simulink model "gm_hybrid_lht"  (R2019b)
settings: Solver=FixedStepDiscrete  StartTime=0.0  StopTime=inf  FixedStep=1/120e6  RelTol=1e-3
undefined symbols (not defined in the file or in its folder): bt, height, nTheta, width
libraries: hdlsllib x42, simulink x32, hdlmdlgenlib x7, dspsrcs4 x1
(part 3 of 3)

== system gm_hybrid_lht/Hybrid LHT/Hybrid LHT Accumulator/Accumulator with Switches/Accumulator_instance2/Block RAM/Simple Dual Port RAM Generator ==
  wr_data : Inport  OutDataTypeStr=fixdt(0, 36, 0)  PortDimensions=1  SampleTime=8.33333333333333e-09
  wr_addr : Inport  Port=2  OutDataTypeStr=fixdt(0, 10, 0)  PortDimensions=1  SampleTime=8.33333333333333e-09
  wr_en : Inport  Port=3  OutDataTypeStr=boolean  PortDimensions=1  SampleTime=8.33333333333333e-09
  rd_addr : Inport  Port=4  OutDataTypeStr=fixdt(0, 10, 0)  PortDimensions=1  SampleTime=8.33333333333333e-09
  rd_address : hdlsllib/Logic and Bit Operations/Bit Slice  lidx=9  ridx=0
      settings: SourceProductName=Simulink  SourceProductBaseCode=SL
  simple_ram_0 : hdlsllib/HDL RAMs/Simple Dual Port RAM  ram_size=10
      settings: SourceProductName=Simulink  SourceProductBaseCode=SL
  wr_address : hdlsllib/Logic and Bit Operations/Bit Slice  lidx=9  ridx=0
      settings: SourceProductName=Simulink  SourceProductBaseCode=SL
  rd_data : Outport
  wires:
  rd_addr/1 -> rd_address/1
  wr_en/1 -> simple_ram_0/3
  wr_addr/1 -> wr_address/1
  wr_data/1 -> simple_ram_0/1
  rd_address/1 -> simple_ram_0/4
  simple_ram_0/1 -> rd_data/1
  wr_address/1 -> simple_ram_0/2

== system gm_hybrid_lht/Hybrid LHT/Hybrid LHT Accumulator/Accumulator with Switches/Accumulator_instance3/Block RAM/Simple Dual Port RAM Generator ==
  wr_data : Inport  OutDataTypeStr=fixdt(0, 36, 0)  PortDimensions=1  SampleTime=8.33333333333333e-09
  wr_addr : Inport  Port=2  OutDataTypeStr=fixdt(0, 10, 0)  PortDimensions=1  SampleTime=8.33333333333333e-09
  wr_en : Inport  Port=3  OutDataTypeStr=boolean  PortDimensions=1  SampleTime=8.33333333333333e-09
  rd_addr : Inport  Port=4  OutDataTypeStr=fixdt(0, 10, 0)  PortDimensions=1  SampleTime=8.33333333333333e-09
  rd_address : hdlsllib/Logic and Bit Operations/Bit Slice  lidx=9  ridx=0
      settings: SourceProductName=Simulink  SourceProductBaseCode=SL
  simple_ram_0 : hdlsllib/HDL RAMs/Simple Dual Port RAM  ram_size=10
      settings: SourceProductName=Simulink  SourceProductBaseCode=SL
  wr_address : hdlsllib/Logic and Bit Operations/Bit Slice  lidx=9  ridx=0
      settings: SourceProductName=Simulink  SourceProductBaseCode=SL
  rd_data : Outport
  wires:
  rd_addr/1 -> rd_address/1
  wr_en/1 -> simple_ram_0/3
  wr_addr/1 -> wr_address/1
  wr_data/1 -> simple_ram_0/1
  rd_address/1 -> simple_ram_0/4
  simple_ram_0/1 -> rd_data/1
  wr_address/1 -> simple_ram_0/2

== system gm_hybrid_lht/Hybrid LHT/Hybrid LHT Accumulator/Accumulator with Switches/Accumulator_instance4/Block RAM/Simple Dual Port RAM Generator ==
  wr_data : Inport  OutDataTypeStr=fixdt(0, 36, 0)  PortDimensions=1  SampleTime=8.33333333333333e-09
  wr_addr : Inport  Port=2  OutDataTypeStr=fixdt(0, 10, 0)  PortDimensions=1  SampleTime=8.33333333333333e-09
  wr_en : Inport  Port=3  OutDataTypeStr=boolean  PortDimensions=1  SampleTime=8.33333333333333e-09
  rd_addr : Inport  Port=4  OutDataTypeStr=fixdt(0, 10, 0)  PortDimensions=1  SampleTime=8.33333333333333e-09
  rd_address : hdlsllib/Logic and Bit Operations/Bit Slice  lidx=9  ridx=0
      settings: SourceProductName=Simulink  SourceProductBaseCode=SL
  simple_ram_0 : hdlsllib/HDL RAMs/Simple Dual Port RAM  ram_size=10
      settings: SourceProductName=Simulink  SourceProductBaseCode=SL
  wr_address : hdlsllib/Logic and Bit Operations/Bit Slice  lidx=9  ridx=0
      settings: SourceProductName=Simulink  SourceProductBaseCode=SL
  rd_data : Outport
  wires:
  rd_addr/1 -> rd_address/1
  wr_en/1 -> simple_ram_0/3
  wr_addr/1 -> wr_address/1
  wr_data/1 -> simple_ram_0/1
  rd_address/1 -> simple_ram_0/4
  simple_ram_0/1 -> rd_data/1
  wr_address/1 -> simple_ram_0/2

== system gm_hybrid_lht/Hybrid LHT/Hybrid LHT Accumulator/Accumulator with Switches/Accumulator_instance5/Block RAM/Simple Dual Port RAM Generator ==
  wr_data : Inport  OutDataTypeStr=fixdt(0, 36, 0)  PortDimensions=1  SampleTime=8.33333333333333e-09
  wr_addr : Inport  Port=2  OutDataTypeStr=fixdt(0, 10, 0)  PortDimensions=1  SampleTime=8.33333333333333e-09
  wr_en : Inport  Port=3  OutDataTypeStr=boolean  PortDimensions=1  SampleTime=8.33333333333333e-09
  rd_addr : Inport  Port=4  OutDataTypeStr=fixdt(0, 10, 0)  PortDimensions=1  SampleTime=8.33333333333333e-09
  rd_address : hdlsllib/Logic and Bit Operations/Bit Slice  lidx=9  ridx=0
      settings: SourceProductName=Simulink  SourceProductBaseCode=SL
  simple_ram_0 : hdlsllib/HDL RAMs/Simple Dual Port RAM  ram_size=10
      settings: SourceProductName=Simulink  SourceProductBaseCode=SL
  wr_address : hdlsllib/Logic and Bit Operations/Bit Slice  lidx=9  ridx=0
      settings: SourceProductName=Simulink  SourceProductBaseCode=SL
  rd_data : Outport
  wires:
  rd_addr/1 -> rd_address/1
  wr_en/1 -> simple_ram_0/3
  wr_addr/1 -> wr_address/1
  wr_data/1 -> simple_ram_0/1
  rd_address/1 -> simple_ram_0/4
  simple_ram_0/1 -> rd_data/1
  wr_address/1 -> simple_ram_0/2

== system gm_hybrid_lht/Hybrid LHT/Hybrid LHT Accumulator/Accumulator with Switches/Accumulator_instance6/Block RAM/Simple Dual Port RAM Generator ==
  wr_data : Inport  OutDataTypeStr=fixdt(0, 36, 0)  PortDimensions=1  SampleTime=8.33333333333333e-09
  wr_addr : Inport  Port=2  OutDataTypeStr=fixdt(0, 10, 0)  PortDimensions=1  SampleTime=8.33333333333333e-09
  wr_en : Inport  Port=3  OutDataTypeStr=boolean  PortDimensions=1  SampleTime=8.33333333333333e-09
  rd_addr : Inport  Port=4  OutDataTypeStr=fixdt(0, 10, 0)  PortDimensions=1  SampleTime=8.33333333333333e-09
  rd_address : hdlsllib/Logic and Bit Operations/Bit Slice  lidx=9  ridx=0
      settings: SourceProductName=Simulink  SourceProductBaseCode=SL
  simple_ram_0 : hdlsllib/HDL RAMs/Simple Dual Port RAM  ram_size=10
      settings: SourceProductName=Simulink  SourceProductBaseCode=SL
  wr_address : hdlsllib/Logic and Bit Operations/Bit Slice  lidx=9  ridx=0
      settings: SourceProductName=Simulink  SourceProductBaseCode=SL
  rd_data : Outport
  wires:
  rd_addr/1 -> rd_address/1
  wr_en/1 -> simple_ram_0/3
  wr_addr/1 -> wr_address/1
  wr_data/1 -> simple_ram_0/1
  rd_address/1 -> simple_ram_0/4
  simple_ram_0/1 -> rd_data/1
  wr_address/1 -> simple_ram_0/2

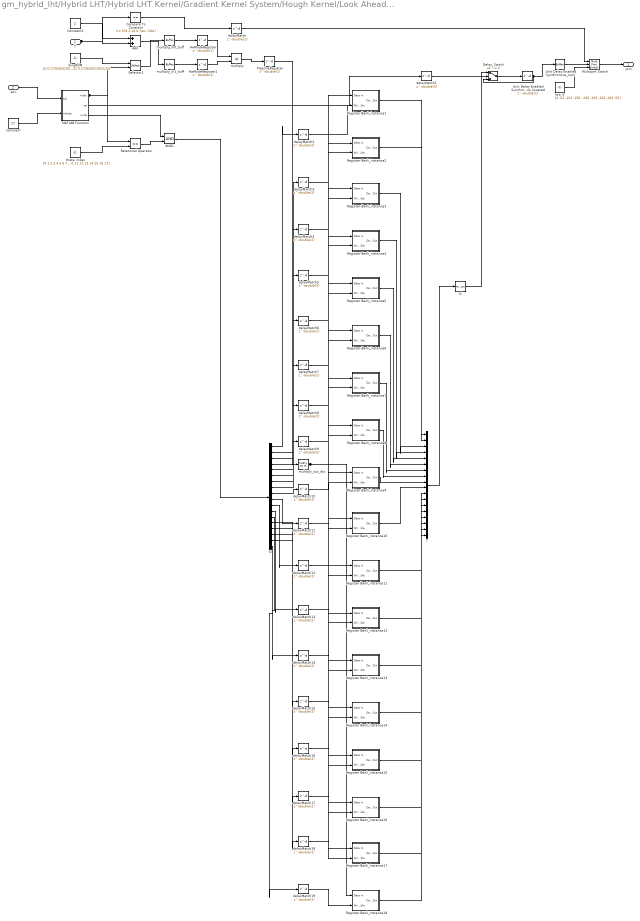
== system gm_hybrid_lht/Hybrid LHT/Hybrid LHT Kernel/Gradient Kernel System/Hough Kernel/Look Ahead Hough/Look Ahead Hough ==
  Y : Inport  OutDataTypeStr=fixdt(1, 10, 0)  PortDimensions=1  SampleTime=8.33333333333333e-09
  eol : Inport  Port=2  OutDataTypeStr=boolean  PortDimensions=1  SampleTime=8.33333333333333e-09
  AND1 : Logic  AllPortsSameDT=off  OutDataTypeStr=boolean  SampleTime=8.33333333333333e-09
  Add : Sum  AccumDataTypeStr=fixdt(1, 11, 0)  OutDataTypeStr=fixdt(1, 10, 0)  SampleTime=8.33333333333333e-09
  Compare To Constant : simulink/Logic and Bit Operations/Compare To Constant  relop===  const=fi(0,1,10,0,'hex','2d4')  OutDataTypeStr=boolean
  Constant : Constant  Value=17  OutDataTypeStr=fixdt(0, 5, 0)  SampleTime=-1
  Constant1 : Constant  OutDataTypeStr=fixdt(1, 10, 0)  SampleTime=-1
  Delay_Switch : Switch  Criteria=u2 ~= 0  Threshold=double(0)  OutDataTypeStr=fixdt(1, 10, 0)  SampleTime=8.33333333333333e-09
  HwModeRegister : Delay  DelayLength=double(1)  InitialCondition=0  SampleTime=8.33333333333333e-09
  HwModeRegister1 : Delay  DelayLength=double(1)  InitialCondition=0  SampleTime=8.33333333333333e-09
  MATLAB Function : Subsystem
  Multiport Switch : MultiPortSwitch  DataPortOrder=Zero-based contiguous  Inputs=2  DiagnosticForDefault=None  zeroidx=on  OutDataTypeStr=fixdt(1, 10, 0)  SampleTime=8.33333333333333e-09
  PipelineRegister : Delay  DelayLength=double(1)  InitialCondition=0  SampleTime=8.33333333333333e-09
  Register Bank_instance1 : Subsystem
  Register Bank_instance10 : Subsystem
  Register Bank_instance11 : Subsystem
  Register Bank_instance12 : Subsystem
  Register Bank_instance13 : Subsystem
  Register Bank_instance14 : Subsystem
  Register Bank_instance15 : Subsystem
  Register Bank_instance16 : Subsystem
  Register Bank_instance17 : Subsystem
  Register Bank_instance18 : Subsystem
  Register Bank_instance2 : Subsystem
  Register Bank_instance3 : Subsystem
  Register Bank_instance4 : Subsystem
  Register Bank_instance5 : Subsystem
  Register Bank_instance6 : Subsystem
  Register Bank_instance7 : Subsystem
  Register Bank_instance8 : Subsystem
  Register Bank_instance9 : Subsystem
  Relational Operator : RelationalOperator  Operator===  OutDataTypeStr=boolean  SampleTime=8.33333333333333e-09  RndMeth=Nearest
  Selector1 : Selector  NumberOfDimensions=2  IndexMode=Zero-based  SampleTime=8.33333333333333e-09  IndexOptions=Index vector (dialog),Index vector (port)  Indices=double(0),double(1)  OutputSizes=double(1),double(1)
  SineROM : Constant  Value=[0 0.17364501953125 0.342041015625 0.5 0.64276123046875 0.76605224609375 0.86602783203125 0.939697265625 0.98480224609375 1 0.98480224609375 0.939697265625 0.86602783203125 0.76605224609375 0.64276123046875 0.5 0.342041015625 0.17364501953125]  VectorParams1D=off  OutDataTypeStr=fixdt(1, 16, 14)  SampleTime=-1
  Unit Delay Enabled Synchronous_lowered : Delay  DelayLength=double(1)  InitialCondition=0  SampleTime=8.33333333333333e-09
  Unit Delay Enabled Synchronous_out1 : hdlmdlgenlib/Buffer
      settings: SourceProductName=Simulink  SourceProductBaseCode=SL
  delayMatch{,1..19} (20 alike) : Delay  DelayLength=double(2)  InitialCondition=0  SampleTime=8.33333333333333e-09
  multiply : Product  Inputs=**  OutDataTypeStr=fixdt(1, 26, 14)  SampleTime=8.33333333333333e-09
  multiply_in0_buff : hdlmdlgenlib/Buffer
      settings: SourceProductName=Simulink  SourceProductBaseCode=SL
  multiply_in1_buff : hdlmdlgenlib/Buffer
      settings: SourceProductName=Simulink  SourceProductBaseCode=SL
  multiply_out_dtc : DataTypeConversion  OutDataTypeStr=fixdt(1, 10, 0)  RndMeth=Round  SampleTime=8.33333333333333e-09
  row_0 : Constant  Value=[0 -52 -103 -150 -193 -230 -260 -282 -295 -300 -295 -282 -260 -230 -193 -150 -103 -52]  VectorParams1D=off  OutDataTypeStr=fixdt(1, 10, 0)  SampleTime=-1
  t : Concatenate  NumInputs=18
  t1 : Reshape  OutputDimensionality=Row vector (2-D)
  t2 : Demux  Outputs=18
  theta_index : Constant  Value=[0 1 2 3 4 5 6 7 8 9 10 11 12 13 14 15 16 17]  VectorParams1D=off  OutDataTypeStr=uint8  SampleTime=-1
  ysin : Outport  VectorParamsAs1DForOutWhenUnconnected=off
  wires:
  Constant/1 -> MATLAB Function/2(ntheta)
  Constant1/1 -> Add/1
  MATLAB Function/1(index) -> Relational Operator/1, Selector1/2
  MATLAB Function/3(write) -> AND1/1
  Multiport Switch/1 -> ysin/1
  Relational Operator/1 -> AND1/2
  SineROM/1 -> Selector1/1
  row_0/1 -> Multiport Switch/3
  theta_index/1 -> Relational Operator/2
  Y/1 -> Add/2, Compare To Constant/1
  eol/1 -> MATLAB Function/1(eol)
  MATLAB Function/2(sel) -> delayMatch1/1
  Compare To Constant/1 -> delayMatch/1
  delayMatch/1 -> Multiport Switch/1
  Unit Delay Enabled Synchronous_out1/1 -> Multiport Switch/2
  Unit Delay Enabled Synchronous_lowered/1 -> Delay_Switch/3, Unit Delay Enabled Synchronous_out1/1
  delayMatch1/1 -> Delay_Switch/2
  Delay_Switch/1 -> Unit Delay Enabled Synchronous_lowered/1
  t1/1 -> Delay_Switch/1
  delayMatch2/1 -> Register Bank_instance1/2(Write Enable)
  delayMatch3/1 -> Register Bank_instance2/2(Write Enable)
  Register Bank_instance3/1(Data Out) -> t/3
  delayMatch4/1 -> Register Bank_instance3/2(Write Enable)
  Register Bank_instance4/1(Data Out) -> t/4
  delayMatch5/1 -> Register Bank_instance4/2(Write Enable)
  Register Bank_instance5/1(Data Out) -> t/5
  delayMatch6/1 -> Register Bank_instance5/2(Write Enable)
  Register Bank_instance6/1(Data Out) -> t/6
  delayMatch7/1 -> Register Bank_instance6/2(Write Enable)
  Register Bank_instance7/1(Data Out) -> t/7
  delayMatch8/1 -> Register Bank_instance7/2(Write Enable)
  Register Bank_instance8/1(Data Out) -> t/8
  delayMatch9/1 -> Register Bank_instance8/2(Write Enable)
  Register Bank_instance9/1(Data Out) -> t/9
  delayMatch10/1 -> Register Bank_instance9/2(Write Enable)
  Register Bank_instance10/1(Data Out) -> t/10
  delayMatch11/1 -> Register Bank_instance10/2(Write Enable)
  Register Bank_instance11/1(Data Out) -> t/11
  delayMatch12/1 -> Register Bank_instance11/2(Write Enable)
  Register Bank_instance12/1(Data Out) -> t/12
  delayMatch13/1 -> Register Bank_instance12/2(Write Enable)
  Register Bank_instance13/1(Data Out) -> t/13
  delayMatch14/1 -> Register Bank_instance13/2(Write Enable)
  Register Bank_instance14/1(Data Out) -> t/14
  delayMatch15/1 -> Register Bank_instance14/2(Write Enable)
  Register Bank_instance15/1(Data Out) -> t/15
  delayMatch16/1 -> Register Bank_instance15/2(Write Enable)
  Register Bank_instance16/1(Data Out) -> t/16
  delayMatch17/1 -> Register Bank_instance16/2(Write Enable)
  Register Bank_instance17/1(Data Out) -> t/17
  delayMatch18/1 -> Register Bank_instance17/2(Write Enable)
  AND1/1 -> t2/1
  t2/1 -> delayMatch2/1
  t2/2 -> delayMatch3/1
  t2/3 -> delayMatch4/1
  t2/4 -> delayMatch5/1
  t2/5 -> delayMatch6/1
  t2/6 -> delayMatch7/1
  t2/7 -> delayMatch8/1
  t2/8 -> delayMatch9/1
  t2/9 -> delayMatch10/1
  t2/10 -> delayMatch11/1
  t2/11 -> delayMatch12/1
  t2/12 -> delayMatch13/1
  t2/13 -> delayMatch14/1
  t2/14 -> delayMatch15/1
  t2/15 -> delayMatch16/1
  t2/16 -> delayMatch17/1
  t2/17 -> delayMatch18/1
  t2/18 -> delayMatch19/1
  delayMatch19/1 -> Register Bank_instance18/2(Write Enable)
  Register Bank_instance18/1(Data Out) -> t/18
  Selector1/1 -> multiply_in0_buff/1
  Add/1 -> multiply_in1_buff/1
  PipelineRegister/1 -> multiply_out_dtc/1
  multiply_out_dtc/1 -> Register Bank_instance18/1(Data In), Register Bank_instance17/1(Data In), Register Bank_instance16/1(Data In), Register Bank_instance15/1(Data In), Register Bank_instance14/1(Data In), Register Bank_instance13/1(Data In), Register Bank_instance12/1(Data In), Register Bank_instance11/1(Data In), Register Bank_instance10/1(Data In), Register Bank_instance9/1(Data In), Register Bank_instance8/1(Data In), Register Bank_instance7/1(Data In), Register Bank_instance6/1(Data In), Register Bank_instance5/1(Data In), Register Bank_instance4/1(Data In), Register Bank_instance3/1(Data In), Register Bank_instance2/1(Data In), Register Bank_instance1/1(Data In)
  Register Bank_instance2/1(Data Out) -> t/2
  Register Bank_instance1/1(Data Out) -> t/1
  t/1 -> t1/1
  multiply/1 -> PipelineRegister/1
  HwModeRegister/1 -> multiply/1
  HwModeRegister1/1 -> multiply/2
  multiply_in0_buff/1 -> HwModeRegister/1
  multiply_in1_buff/1 -> HwModeRegister1/1

== system gm_hybrid_lht/Hybrid LHT/Hybrid LHT Kernel/Gradient Kernel System/Hough Kernel/Look Ahead Hough/Look Ahead Hough/MATLAB Function ==
  eol : Inport  OutDataTypeStr=boolean  PortDimensions=1  SampleTime=8.33333333333333e-09
  ntheta : Inport  Port=2  OutDataTypeStr=fixdt(0, 5, 0)  PortDimensions=1  SampleTime=8.33333333333333e-09
  MATLAB Function : MATLAB Function  TreatAsAtomicUnit=on
  index : Outport  VectorParamsAs1DForOutWhenUnconnected=off
  sel : Outport  Port=2  VectorParamsAs1DForOutWhenUnconnected=off
  write : Outport  Port=3  VectorParamsAs1DForOutWhenUnconnected=off
  wires:
  MATLAB Function/1(index) -> index/1
  MATLAB Function/2(sel) -> sel/1
  MATLAB Function/3(write) -> write/1
  eol/1 -> MATLAB Function/1(eol)
  ntheta/1 -> MATLAB Function/2(ntheta)

== system gm_hybrid_lht/Hybrid LHT/Hybrid LHT Kernel/Gradient Kernel System/Hough Kernel/Look Ahead Hough/Look Ahead Hough/Register Bank_instance1 ==
  Data In : Inport  OutDataTypeStr=fixdt(1, 10, 0)  PortDimensions=1  SampleTime=8.33333333333333e-09
  Write Enable : Inport  Port=2  OutDataTypeStr=boolean  PortDimensions=1  SampleTime=8.33333333333333e-09
  Delay_Switch : Switch  Criteria=u2 ~= 0  Threshold=double(0)  OutDataTypeStr=fixdt(1, 10, 0)  SampleTime=8.33333333333333e-09
  Unit Delay Enabled Synchronous_lowered : Delay  DelayLength=double(1)  InitialCondition=0  SampleTime=8.33333333333333e-09
  Data Out : Outport
  wires:
  Delay_Switch/1 -> Unit Delay Enabled Synchronous_lowered/1
  Write Enable/1 -> Delay_Switch/2
  Data In/1 -> Delay_Switch/1
  Unit Delay Enabled Synchronous_lowered/1 -> Delay_Switch/3, Data Out/1

== system gm_hybrid_lht/Hybrid LHT/Hybrid LHT Kernel/Gradient Kernel System/Hough Kernel/Look Ahead Hough/Look Ahead Hough/Register Bank_instance10 ==
  Data In : Inport  OutDataTypeStr=fixdt(1, 10, 0)  PortDimensions=1  SampleTime=8.33333333333333e-09
  Write Enable : Inport  Port=2  OutDataTypeStr=boolean  PortDimensions=1  SampleTime=8.33333333333333e-09
  Delay_Switch : Switch  Criteria=u2 ~= 0  Threshold=double(0)  OutDataTypeStr=fixdt(1, 10, 0)  SampleTime=8.33333333333333e-09
  Unit Delay Enabled Synchronous_lowered : Delay  DelayLength=double(1)  InitialCondition=0  SampleTime=8.33333333333333e-09
  Data Out : Outport
  wires:
  Delay_Switch/1 -> Unit Delay Enabled Synchronous_lowered/1
  Write Enable/1 -> Delay_Switch/2
  Data In/1 -> Delay_Switch/1
  Unit Delay Enabled Synchronous_lowered/1 -> Delay_Switch/3, Data Out/1

== system gm_hybrid_lht/Hybrid LHT/Hybrid LHT Kernel/Gradient Kernel System/Hough Kernel/Look Ahead Hough/Look Ahead Hough/Register Bank_instance11 ==
  Data In : Inport  OutDataTypeStr=fixdt(1, 10, 0)  PortDimensions=1  SampleTime=8.33333333333333e-09
  Write Enable : Inport  Port=2  OutDataTypeStr=boolean  PortDimensions=1  SampleTime=8.33333333333333e-09
  Delay_Switch : Switch  Criteria=u2 ~= 0  Threshold=double(0)  OutDataTypeStr=fixdt(1, 10, 0)  SampleTime=8.33333333333333e-09
  Unit Delay Enabled Synchronous_lowered : Delay  DelayLength=double(1)  InitialCondition=0  SampleTime=8.33333333333333e-09
  Data Out : Outport
  wires:
  Delay_Switch/1 -> Unit Delay Enabled Synchronous_lowered/1
  Write Enable/1 -> Delay_Switch/2
  Data In/1 -> Delay_Switch/1
  Unit Delay Enabled Synchronous_lowered/1 -> Delay_Switch/3, Data Out/1

== system gm_hybrid_lht/Hybrid LHT/Hybrid LHT Kernel/Gradient Kernel System/Hough Kernel/Look Ahead Hough/Look Ahead Hough/Register Bank_instance12 ==
  Data In : Inport  OutDataTypeStr=fixdt(1, 10, 0)  PortDimensions=1  SampleTime=8.33333333333333e-09
  Write Enable : Inport  Port=2  OutDataTypeStr=boolean  PortDimensions=1  SampleTime=8.33333333333333e-09
  Delay_Switch : Switch  Criteria=u2 ~= 0  Threshold=double(0)  OutDataTypeStr=fixdt(1, 10, 0)  SampleTime=8.33333333333333e-09
  Unit Delay Enabled Synchronous_lowered : Delay  DelayLength=double(1)  InitialCondition=0  SampleTime=8.33333333333333e-09
  Data Out : Outport
  wires:
  Delay_Switch/1 -> Unit Delay Enabled Synchronous_lowered/1
  Write Enable/1 -> Delay_Switch/2
  Data In/1 -> Delay_Switch/1
  Unit Delay Enabled Synchronous_lowered/1 -> Delay_Switch/3, Data Out/1

== system gm_hybrid_lht/Hybrid LHT/Hybrid LHT Kernel/Gradient Kernel System/Hough Kernel/Look Ahead Hough/Look Ahead Hough/Register Bank_instance13 ==
  Data In : Inport  OutDataTypeStr=fixdt(1, 10, 0)  PortDimensions=1  SampleTime=8.33333333333333e-09
  Write Enable : Inport  Port=2  OutDataTypeStr=boolean  PortDimensions=1  SampleTime=8.33333333333333e-09
  Delay_Switch : Switch  Criteria=u2 ~= 0  Threshold=double(0)  OutDataTypeStr=fixdt(1, 10, 0)  SampleTime=8.33333333333333e-09
  Unit Delay Enabled Synchronous_lowered : Delay  DelayLength=double(1)  InitialCondition=0  SampleTime=8.33333333333333e-09
  Data Out : Outport
  wires:
  Delay_Switch/1 -> Unit Delay Enabled Synchronous_lowered/1
  Write Enable/1 -> Delay_Switch/2
  Data In/1 -> Delay_Switch/1
  Unit Delay Enabled Synchronous_lowered/1 -> Delay_Switch/3, Data Out/1

== system gm_hybrid_lht/Hybrid LHT/Hybrid LHT Kernel/Gradient Kernel System/Hough Kernel/Look Ahead Hough/Look Ahead Hough/Register Bank_instance14 ==
  Data In : Inport  OutDataTypeStr=fixdt(1, 10, 0)  PortDimensions=1  SampleTime=8.33333333333333e-09
  Write Enable : Inport  Port=2  OutDataTypeStr=boolean  PortDimensions=1  SampleTime=8.33333333333333e-09
  Delay_Switch : Switch  Criteria=u2 ~= 0  Threshold=double(0)  OutDataTypeStr=fixdt(1, 10, 0)  SampleTime=8.33333333333333e-09
  Unit Delay Enabled Synchronous_lowered : Delay  DelayLength=double(1)  InitialCondition=0  SampleTime=8.33333333333333e-09
  Data Out : Outport
  wires:
  Delay_Switch/1 -> Unit Delay Enabled Synchronous_lowered/1
  Write Enable/1 -> Delay_Switch/2
  Data In/1 -> Delay_Switch/1
  Unit Delay Enabled Synchronous_lowered/1 -> Delay_Switch/3, Data Out/1

== system gm_hybrid_lht/Hybrid LHT/Hybrid LHT Kernel/Gradient Kernel System/Hough Kernel/Look Ahead Hough/Look Ahead Hough/Register Bank_instance15 ==
  Data In : Inport  OutDataTypeStr=fixdt(1, 10, 0)  PortDimensions=1  SampleTime=8.33333333333333e-09
  Write Enable : Inport  Port=2  OutDataTypeStr=boolean  PortDimensions=1  SampleTime=8.33333333333333e-09
  Delay_Switch : Switch  Criteria=u2 ~= 0  Threshold=double(0)  OutDataTypeStr=fixdt(1, 10, 0)  SampleTime=8.33333333333333e-09
  Unit Delay Enabled Synchronous_lowered : Delay  DelayLength=double(1)  InitialCondition=0  SampleTime=8.33333333333333e-09
  Data Out : Outport
  wires:
  Delay_Switch/1 -> Unit Delay Enabled Synchronous_lowered/1
  Write Enable/1 -> Delay_Switch/2
  Data In/1 -> Delay_Switch/1
  Unit Delay Enabled Synchronous_lowered/1 -> Delay_Switch/3, Data Out/1

== system gm_hybrid_lht/Hybrid LHT/Hybrid LHT Kernel/Gradient Kernel System/Hough Kernel/Look Ahead Hough/Look Ahead Hough/Register Bank_instance16 ==
  Data In : Inport  OutDataTypeStr=fixdt(1, 10, 0)  PortDimensions=1  SampleTime=8.33333333333333e-09
  Write Enable : Inport  Port=2  OutDataTypeStr=boolean  PortDimensions=1  SampleTime=8.33333333333333e-09
  Delay_Switch : Switch  Criteria=u2 ~= 0  Threshold=double(0)  OutDataTypeStr=fixdt(1, 10, 0)  SampleTime=8.33333333333333e-09
  Unit Delay Enabled Synchronous_lowered : Delay  DelayLength=double(1)  InitialCondition=0  SampleTime=8.33333333333333e-09
  Data Out : Outport
  wires:
  Delay_Switch/1 -> Unit Delay Enabled Synchronous_lowered/1
  Write Enable/1 -> Delay_Switch/2
  Data In/1 -> Delay_Switch/1
  Unit Delay Enabled Synchronous_lowered/1 -> Delay_Switch/3, Data Out/1

== system gm_hybrid_lht/Hybrid LHT/Hybrid LHT Kernel/Gradient Kernel System/Hough Kernel/Look Ahead Hough/Look Ahead Hough/Register Bank_instance17 ==
  Data In : Inport  OutDataTypeStr=fixdt(1, 10, 0)  PortDimensions=1  SampleTime=8.33333333333333e-09
  Write Enable : Inport  Port=2  OutDataTypeStr=boolean  PortDimensions=1  SampleTime=8.33333333333333e-09
  Delay_Switch : Switch  Criteria=u2 ~= 0  Threshold=double(0)  OutDataTypeStr=fixdt(1, 10, 0)  SampleTime=8.33333333333333e-09
  Unit Delay Enabled Synchronous_lowered : Delay  DelayLength=double(1)  InitialCondition=0  SampleTime=8.33333333333333e-09
  Data Out : Outport
  wires:
  Delay_Switch/1 -> Unit Delay Enabled Synchronous_lowered/1
  Write Enable/1 -> Delay_Switch/2
  Data In/1 -> Delay_Switch/1
  Unit Delay Enabled Synchronous_lowered/1 -> Delay_Switch/3, Data Out/1

== system gm_hybrid_lht/Hybrid LHT/Hybrid LHT Kernel/Gradient Kernel System/Hough Kernel/Look Ahead Hough/Look Ahead Hough/Register Bank_instance18 ==
  Data In : Inport  OutDataTypeStr=fixdt(1, 10, 0)  PortDimensions=1  SampleTime=8.33333333333333e-09
  Write Enable : Inport  Port=2  OutDataTypeStr=boolean  PortDimensions=1  SampleTime=8.33333333333333e-09
  Delay_Switch : Switch  Criteria=u2 ~= 0  Threshold=double(0)  OutDataTypeStr=fixdt(1, 10, 0)  SampleTime=8.33333333333333e-09
  Unit Delay Enabled Synchronous_lowered : Delay  DelayLength=double(1)  InitialCondition=0  SampleTime=8.33333333333333e-09
  Data Out : Outport
  wires:
  Delay_Switch/1 -> Unit Delay Enabled Synchronous_lowered/1
  Write Enable/1 -> Delay_Switch/2
  Data In/1 -> Delay_Switch/1
  Unit Delay Enabled Synchronous_lowered/1 -> Delay_Switch/3, Data Out/1

== system gm_hybrid_lht/Hybrid LHT/Hybrid LHT Kernel/Gradient Kernel System/Hough Kernel/Look Ahead Hough/Look Ahead Hough/Register Bank_instance2 ==
  Data In : Inport  OutDataTypeStr=fixdt(1, 10, 0)  PortDimensions=1  SampleTime=8.33333333333333e-09
  Write Enable : Inport  Port=2  OutDataTypeStr=boolean  PortDimensions=1  SampleTime=8.33333333333333e-09
  Delay_Switch : Switch  Criteria=u2 ~= 0  Threshold=double(0)  OutDataTypeStr=fixdt(1, 10, 0)  SampleTime=8.33333333333333e-09
  Unit Delay Enabled Synchronous_lowered : Delay  DelayLength=double(1)  InitialCondition=0  SampleTime=8.33333333333333e-09
  Data Out : Outport
  wires:
  Delay_Switch/1 -> Unit Delay Enabled Synchronous_lowered/1
  Write Enable/1 -> Delay_Switch/2
  Data In/1 -> Delay_Switch/1
  Unit Delay Enabled Synchronous_lowered/1 -> Delay_Switch/3, Data Out/1

== system gm_hybrid_lht/Hybrid LHT/Hybrid LHT Kernel/Gradient Kernel System/Hough Kernel/Look Ahead Hough/Look Ahead Hough/Register Bank_instance3 ==
  Data In : Inport  OutDataTypeStr=fixdt(1, 10, 0)  PortDimensions=1  SampleTime=8.33333333333333e-09
  Write Enable : Inport  Port=2  OutDataTypeStr=boolean  PortDimensions=1  SampleTime=8.33333333333333e-09
  Delay_Switch : Switch  Criteria=u2 ~= 0  Threshold=double(0)  OutDataTypeStr=fixdt(1, 10, 0)  SampleTime=8.33333333333333e-09
  Unit Delay Enabled Synchronous_lowered : Delay  DelayLength=double(1)  InitialCondition=0  SampleTime=8.33333333333333e-09
  Data Out : Outport
  wires:
  Unit Delay Enabled Synchronous_lowered/1 -> Data Out/1, Delay_Switch/3
  Data In/1 -> Delay_Switch/1
  Write Enable/1 -> Delay_Switch/2
  Delay_Switch/1 -> Unit Delay Enabled Synchronous_lowered/1

== system gm_hybrid_lht/Hybrid LHT/Hybrid LHT Kernel/Gradient Kernel System/Hough Kernel/Look Ahead Hough/Look Ahead Hough/Register Bank_instance4 ==
  Data In : Inport  OutDataTypeStr=fixdt(1, 10, 0)  PortDimensions=1  SampleTime=8.33333333333333e-09
  Write Enable : Inport  Port=2  OutDataTypeStr=boolean  PortDimensions=1  SampleTime=8.33333333333333e-09
  Delay_Switch : Switch  Criteria=u2 ~= 0  Threshold=double(0)  OutDataTypeStr=fixdt(1, 10, 0)  SampleTime=8.33333333333333e-09
  Unit Delay Enabled Synchronous_lowered : Delay  DelayLength=double(1)  InitialCondition=0  SampleTime=8.33333333333333e-09
  Data Out : Outport
  wires:
  Delay_Switch/1 -> Unit Delay Enabled Synchronous_lowered/1
  Write Enable/1 -> Delay_Switch/2
  Data In/1 -> Delay_Switch/1
  Unit Delay Enabled Synchronous_lowered/1 -> Delay_Switch/3, Data Out/1

== system gm_hybrid_lht/Hybrid LHT/Hybrid LHT Kernel/Gradient Kernel System/Hough Kernel/Look Ahead Hough/Look Ahead Hough/Register Bank_instance5 ==
  Data In : Inport  OutDataTypeStr=fixdt(1, 10, 0)  PortDimensions=1  SampleTime=8.33333333333333e-09
  Write Enable : Inport  Port=2  OutDataTypeStr=boolean  PortDimensions=1  SampleTime=8.33333333333333e-09
  Delay_Switch : Switch  Criteria=u2 ~= 0  Threshold=double(0)  OutDataTypeStr=fixdt(1, 10, 0)  SampleTime=8.33333333333333e-09
  Unit Delay Enabled Synchronous_lowered : Delay  DelayLength=double(1)  InitialCondition=0  SampleTime=8.33333333333333e-09
  Data Out : Outport
  wires:
  Delay_Switch/1 -> Unit Delay Enabled Synchronous_lowered/1
  Write Enable/1 -> Delay_Switch/2
  Data In/1 -> Delay_Switch/1
  Unit Delay Enabled Synchronous_lowered/1 -> Delay_Switch/3, Data Out/1

== system gm_hybrid_lht/Hybrid LHT/Hybrid LHT Kernel/Gradient Kernel System/Hough Kernel/Look Ahead Hough/Look Ahead Hough/Register Bank_instance6 ==
  Data In : Inport  OutDataTypeStr=fixdt(1, 10, 0)  PortDimensions=1  SampleTime=8.33333333333333e-09
  Write Enable : Inport  Port=2  OutDataTypeStr=boolean  PortDimensions=1  SampleTime=8.33333333333333e-09
  Delay_Switch : Switch  Criteria=u2 ~= 0  Threshold=double(0)  OutDataTypeStr=fixdt(1, 10, 0)  SampleTime=8.33333333333333e-09
  Unit Delay Enabled Synchronous_lowered : Delay  DelayLength=double(1)  InitialCondition=0  SampleTime=8.33333333333333e-09
  Data Out : Outport
  wires:
  Delay_Switch/1 -> Unit Delay Enabled Synchronous_lowered/1
  Write Enable/1 -> Delay_Switch/2
  Data In/1 -> Delay_Switch/1
  Unit Delay Enabled Synchronous_lowered/1 -> Delay_Switch/3, Data Out/1

== system gm_hybrid_lht/Hybrid LHT/Hybrid LHT Kernel/Gradient Kernel System/Hough Kernel/Look Ahead Hough/Look Ahead Hough/Register Bank_instance7 ==
  Data In : Inport  OutDataTypeStr=fixdt(1, 10, 0)  PortDimensions=1  SampleTime=8.33333333333333e-09
  Write Enable : Inport  Port=2  OutDataTypeStr=boolean  PortDimensions=1  SampleTime=8.33333333333333e-09
  Delay_Switch : Switch  Criteria=u2 ~= 0  Threshold=double(0)  OutDataTypeStr=fixdt(1, 10, 0)  SampleTime=8.33333333333333e-09
  Unit Delay Enabled Synchronous_lowered : Delay  DelayLength=double(1)  InitialCondition=0  SampleTime=8.33333333333333e-09
  Data Out : Outport
  wires:
  Delay_Switch/1 -> Unit Delay Enabled Synchronous_lowered/1
  Write Enable/1 -> Delay_Switch/2
  Data In/1 -> Delay_Switch/1
  Unit Delay Enabled Synchronous_lowered/1 -> Delay_Switch/3, Data Out/1

== system gm_hybrid_lht/Hybrid LHT/Hybrid LHT Kernel/Gradient Kernel System/Hough Kernel/Look Ahead Hough/Look Ahead Hough/Register Bank_instance8 ==
  Data In : Inport  OutDataTypeStr=fixdt(1, 10, 0)  PortDimensions=1  SampleTime=8.33333333333333e-09
  Write Enable : Inport  Port=2  OutDataTypeStr=boolean  PortDimensions=1  SampleTime=8.33333333333333e-09
  Delay_Switch : Switch  Criteria=u2 ~= 0  Threshold=double(0)  OutDataTypeStr=fixdt(1, 10, 0)  SampleTime=8.33333333333333e-09
  Unit Delay Enabled Synchronous_lowered : Delay  DelayLength=double(1)  InitialCondition=0  SampleTime=8.33333333333333e-09
  Data Out : Outport
  wires:
  Delay_Switch/1 -> Unit Delay Enabled Synchronous_lowered/1
  Write Enable/1 -> Delay_Switch/2
  Data In/1 -> Delay_Switch/1
  Unit Delay Enabled Synchronous_lowered/1 -> Delay_Switch/3, Data Out/1

== system gm_hybrid_lht/Hybrid LHT/Hybrid LHT Kernel/Gradient Kernel System/Hough Kernel/Look Ahead Hough/Look Ahead Hough/Register Bank_instance9 ==
  Data In : Inport  OutDataTypeStr=fixdt(1, 10, 0)  PortDimensions=1  SampleTime=8.33333333333333e-09
  Write Enable : Inport  Port=2  OutDataTypeStr=boolean  PortDimensions=1  SampleTime=8.33333333333333e-09
  Delay_Switch : Switch  Criteria=u2 ~= 0  Threshold=double(0)  OutDataTypeStr=fixdt(1, 10, 0)  SampleTime=8.33333333333333e-09
  Unit Delay Enabled Synchronous_lowered : Delay  DelayLength=double(1)  InitialCondition=0  SampleTime=8.33333333333333e-09
  Data Out : Outport
  wires:
  Delay_Switch/1 -> Unit Delay Enabled Synchronous_lowered/1
  Write Enable/1 -> Delay_Switch/2
  Data In/1 -> Delay_Switch/1
  Unit Delay Enabled Synchronous_lowered/1 -> Delay_Switch/3, Data Out/1

== matlab function gm_hybrid_lht/Hybrid LHT/Hybrid LHT Accumulator/Accumulator Controller/Accumulator Controller ==
  data: shift output; sof input; mode output; eof input; read output; clear output; index output; ntheta input; nrho input; valid output; nshift input
function [shift, mode, read, clear, index, valid] = fcn(sof, eof, ntheta, nrho, nshift)

IDLE = fi(0, 0, 2, 0);
VOTE = fi(1, 0, 2, 0);
READ = fi(2, 0, 2, 0);
CLEAR = fi(3, 0, 2, 0);

persistent current_state;
persistent rho_counter;
persistent theta_counter;
persistent shift_counter;

if isempty(current_state)
    current_state = IDLE;
end

if isempty(rho_counter)
    rho_counter = fi(0, 0, 16, 0);
end

if isempty(theta_counter)
    theta_counter = fi(0, 0, 16, 0);
end

if isempty(shift_counter)
    shift_counter = fi(0, 0, 16, 0);
end

switch current_state
    case IDLE
        rho_counter = fi(0, 0, 16, 0);
        theta_counter = fi(0, 0, 16, 0);
        shift_counter = fi(0, 0, 16, 0);
        
        clear = false;
        valid = false;
        
        read = rho_counter;
        index = theta_counter;
        shift = shift_counter;
        
        if sof
            mode = true;
            current_state = VOTE;
        else
            mode = false;
            current_state = IDLE;
        end
        
    case VOTE
        rho_counter = fi(0, 0, 16, 0);
        theta_counter = fi(0, 0, 16, 0);
        shift_counter = fi(0, 0, 16, 0);
        
        mode = true;
        clear = false;
        valid = false;
        
        shift = shift_counter;
        read = rho_counter;
        index = theta_counter;
        
        if eof
            current_state = READ;
        else
            current_state = VOTE;
        end
        
    case READ
        mode = false;
        clear = false;
        valid = true;
        
        read = rho_counter;
        index = theta_counter;
        shift = shift_counter;
        
        if theta_counter >= ntheta && rho_counter >= nrho && shift_counter >= nshift
            rho_counter = fi(0, 0, 16, 0);
            theta_counter = fi(0, 0, 16, 0);
            shift_counter = fi(0, 0, 16, 0);
            current_state = CLEAR;
        elseif theta_counter >= ntheta && rho_counter >= nrho
            theta_counter = fi(0, 0, 16, 0);
            rho_counter = fi(0, 0, 16, 0);
            shift_counter = fi(shift_counter + 1, 0, 16, 0);
            current_state = READ;
        elseif rho_counter >= nrho
            rho_counter = fi(0, 0, 16, 0);
            theta_counter = fi(theta_counter + 1, 0, 16, 0);
            current_state = READ;
        else
            rho_counter = fi(rho_counter + 1, 0, 16, 0);
            current_state = READ;
        end
        
    case CLEAR
        mode = false;
        clear = true;
        valid = false;
        
        read = rho_counter;
        index = theta_counter;
        shift = shift_counter;
        
        if rho_counter >= nrho
            rho_counter = fi(0, 0, 16, 0);
            theta_counter = fi(0, 0, 16, 0);
            shift_counter = fi(0, 0, 16, 0);
            current_state = IDLE;
        else
            rho_counter = fi(rho_counter + 1, 0, 16, 0);
            theta_counter = fi(0, 0, 16, 0);
            shift_counter = fi(0, 0, 16, 0);
            current_state = CLEAR;
        end
        
    otherwise
        rho_counter = fi(0, 0, 16, 0);
        theta_counter = fi(0, 0, 16, 0);
        shift_counter = fi(0, 0, 16, 0);
        
        mode = false;
        clear = false;
        valid = false;
        
        shift = shift_counter;
        read = rho_counter;
        index = theta_counter;
        
        current_state = IDLE;
        
end

== matlab function gm_hybrid_lht/Hybrid LHT/Hybrid LHT Kernel/Gradient Kernel System/Hough Kernel/Look Ahead Hough/Look Ahead Hough/MATLAB Function/MATLAB Function ==
  data: index output; eol input; sel output; write output; ntheta input; debug_state output
function [index, sel, write, debug_state] = fcn(eol, ntheta)

BANK = fi(1, 0, 3, 0);
WAIT = fi(2, 0, 3, 0);

persistent state;

persistent thetacounter;

if isempty(state)
    state = BANK;
end

if isempty(thetacounter)
    thetacounter = fi(0, 0, 16, 0);
end

switch state
    case BANK
        sel = false;
        write = true;
        index = thetacounter;
        debug_state = state;
        
        if thetacounter == ntheta
            thetacounter = fi(0, 0, 16, 0);
            state = WAIT;
        else
            thetacounter = fi(thetacounter + 1, 0, 16, 0);
            state = BANK;
        end
        
    case WAIT
        write = false;
        index = thetacounter;
        debug_state = state;
        
        thetacounter = fi(0, 0, 16, 0);
        
        if eol
            sel = true;
            state = BANK;
        else
            sel = false;
            state = WAIT;
        end
        
    otherwise
        thetacounter = fi(0, 0, 16, 0);
        sel = false;
        write = false;
        index = thetacounter;
        debug_state = state;
        
        state = WAIT;
        
end
